simulink model "Dual_Active_Bridge_Converter"  (R2022b)
settings: Solver=ode23t  StartTime=0.0  StopTime=.1  FixedStep=1e-7  MaxStep=1e-7  RelTol=1e-3
model workspace (MAT data in the model file):
  N_P0 = 3
undefined symbols (not defined in the file or in its folder): Ion, Lithium
libraries: spsIGBTDiodeLib x8, spsCurrentMeasurementLib x3, spsVoltageMeasurementLib x3, spsSeriesRLCBranchLib x2, slpidlib x2, spsBatteryLib x1, spsDCVoltageSourceLib x1, spsLinearTransformerLib x1, dspstat3 x1, sps_lib x1
settings Model: Creator=es-ahmedabdellatif20  LastModifiedBy=es-ahmedabdellatif20

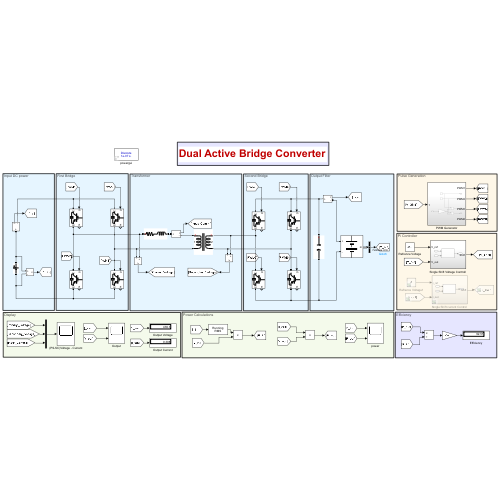
[thumbnail: Simulink's stored preview of the top-level diagram]
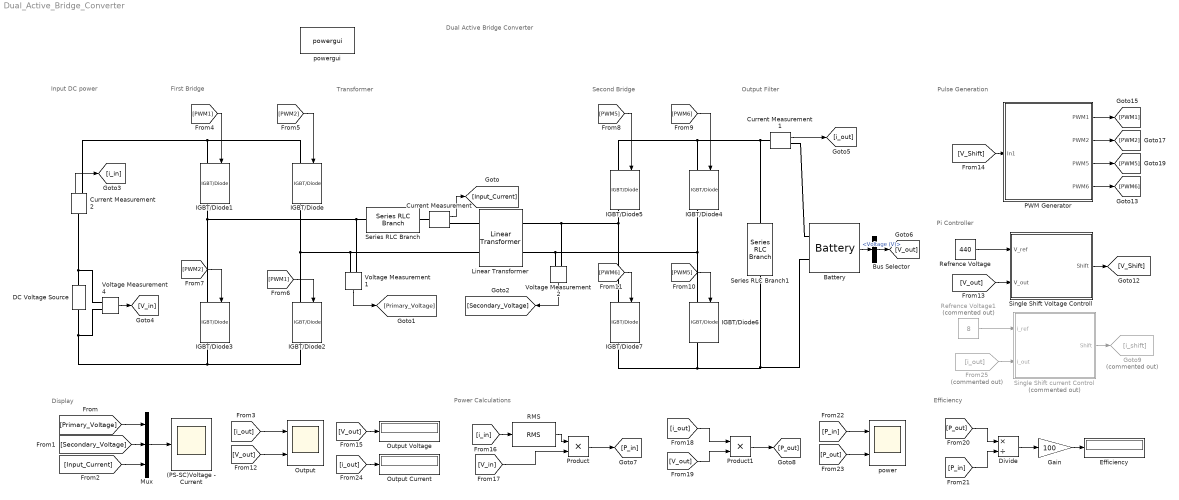
== system Dual_Active_Bridge_Converter ==
  note: Efficiency
  note: Power Calculations
  note: Pi Controller
  note: Pulse Generation
  note: Output Filter
  note: Second Bridge
  note: Transformer
  note: First Bridge
  note: Input DC power
  note: Dual Active Bridge Converter
  note: Display
  (PS-SC)Voltage - Current : Scope
  Battery : spsBatteryLib/Battery  BatType=Lithium-Ion  ShowTempParam=off  ThermalPreset=no  ShowAgeParam=off  NomV=400  NomQ=5  SOC=60  Batt_Tr=30  PresetModel=on  MaxQ=5  MinV=300  FullV=465.5949  Dis_rate=2.1739  R=0.8  Normal_OP=4.5217  expZone="[432.1543     0.2456522]"  current=[6.5 13 32.5]  Units=Time  Tci=20  NomT=20  T2=-30  MaxQ2=4.8  FullV2=7.1  Normal_OP2=5.655  expZone2="[6.58           1]"  Rca=0.6  ti=2000  Dp=0  Neq0=0  Tsim=1e6  Ta1=25  Qeol=5.4*0.9  Reol=0.013333*1.2  Char_age=[2.3478, 3]  Dis_age=[2.3478, 10]  N1=1500  N2=10500  N3=1000  N4=1400  Ta2=45  N5=950
  Bus Selector : BusSelector  OutputSignals=Voltage (V)
  Current Measurement : spsCurrentMeasurementLib/Current Measurement  PhasorSimulation=off  OutputType=Complex  PSBequivalent=0
  Current Measurement1 : spsCurrentMeasurementLib/Current Measurement  PhasorSimulation=off  OutputType=Complex  PSBequivalent=0
  Current Measurement2 : spsCurrentMeasurementLib/Current Measurement  PhasorSimulation=off  OutputType=Complex  PSBequivalent=0
  DC Voltage Source : spsDCVoltageSourceLib/DC Voltage Source  Amplitude=800  Measurements=Voltage
  Divide : Product  Inputs=*/
  Efficiency : Display
  From25 : From  Commented=on  GotoTag=i_out
  Gain : Gain  Gain=100
  Goto9 : Goto  Commented=on  GotoTag=i_shift
  IGBT/Diode{,1..7} (8 alike) : spsIGBTDiodeLib/IGBT//Diode  Ron=1e-3  Rs=1e5  Cs=inf  Measurements=on
  Linear Transformer : spsLinearTransformerLib/Linear Transformer  UNITS=SI  NominalPower=[ 10000 100000 ]  winding1=[800 0 0]  winding2=[450 0 0]  ThreeWindings=off  winding3=[3.15e+05 0.7938 0.084225]  RmLm=[1.0804e+06 2866]  Measurements=None  DataType=on
  Mux : Mux  Inputs=3
  Output : Scope  NumInputPorts=2
  Output Current : Display
  Output Voltage : Display
  PWM Generator : Subsystem
  Product : Product
  Product1 : Product
  RMS : dspstat3/RMS  run=on  directionMode=Each column  dimension=1  InputProcessing=Columns as channels (frame based)  reset_popup=None
  Refrence Voltage : Constant  Value=440
  Refrence Voltage1 : Constant  Commented=on  Value=8
  Series RLC Branch : spsSeriesRLCBranchLib/Series RLC Branch  LConnTagsString=__new0  RConnTagsString=__new0  BranchType=RL  Resistance=.2  Inductance=8.5e-5/2  SetiL0=off  InitialCurrent=5  Capacitance=1e-6  Setx0=off  InitialVoltage=0  Measurements=None
  Series RLC Branch1 : spsSeriesRLCBranchLib/Series RLC Branch  LConnTagsString=__new0  RConnTagsString=__new0  BranchType=C  Resistance=10  Inductance=2.2857e-4  SetiL0=off  InitialCurrent=0  Capacitance=660e-6  Setx0=on  InitialVoltage=250  Measurements=None
  "Single Shift Voltage Controll " : Subsystem
  "Single Shift current Control " : Subsystem  Commented=on
  Voltage Measurement1 : spsVoltageMeasurementLib/Voltage Measurement  PhasorSimulation=off  OutputType=Complex  PSBequivalent=0
  Voltage Measurement2 : spsVoltageMeasurementLib/Voltage Measurement  PhasorSimulation=off  OutputType=Complex  PSBequivalent=0
  Voltage Measurement4 : spsVoltageMeasurementLib/Voltage Measurement  PhasorSimulation=off  OutputType=Complex  PSBequivalent=0
  power : Scope  NumInputPorts=2
  powergui : sps_lib/powergui  Priority=1  SimulationMode=Discrete  SampleTime=1e-7  frequency=60  Iterations=50  frequencyindice=0  Pbase=100e6  ErrMax=1e-4  UnitsV=kV  UnitsW=MW  buscounter=0  FunctionMessages=off  echomessages=off  EnableUseOfTLC=off  CurrentSourceSwitches=off  DisableSnubberDevices=off  DisableRonSwitches=off  DisableVfSwitches=off  DisplayEquations=off  AutomaticDiscreteSolvers=off  SolverType=Tustin/Backward Euler (TBE)  Interpol=off  ExternalGateDelay=off  methode=off  Ts=100  x0status=blocks  SPID=on  SwTol=0  HookPort=off  NonlinearTolerance=1e-4  nMaxIteration=100  ContinueOnMaxIteration=off  RestoreLinks=warning  ResistiveCurrentMeasurement=off  Frange=[0:2:500]  Ylog=off  Xlog=on  ShowGrid=off  save=off  variable=ZData  structure=0  ZoomFFT=off  StartTime=0.0  cycles=1  DisplayStyle=1  fundamental=60  FreqAxis=off  MaxFrequency=1000  frequencyindicesteady=1  RmsSteady=1  display=off
  wires:
  Mux/1 -> (PS-SC)Voltage - Current/1
  Current Measurement/1 -> [Input_Current]
  Voltage Measurement1/1 -> [Primary_Voltage]
  Voltage Measurement2/1 -> [Secondary_Voltage]
  [Primary_Voltage] -> Mux/1
  [Secondary_Voltage] -> Mux/2
  [PWM1] -> IGBT/Diode1/1
  [PWM2] -> IGBT/Diode/1
  [PWM2] -> IGBT/Diode3/1
  [PWM1] -> IGBT/Diode2/1
  [PWM5] -> IGBT/Diode6/1
  [PWM6] -> IGBT/Diode4/1
  [PWM5] -> IGBT/Diode5/1
  [PWM6] -> IGBT/Diode7/1
  PWM Generator/1(PWM1) -> [PWM1]
  PWM Generator/2(PWM2) -> [PWM2]
  PWM Generator/3(PWM5) -> [PWM5]
  PWM Generator/4(PWM6) -> [PWM6]
  [Input_Current] -> Mux/3
  [V_Shift] -> PWM Generator/1(In1)
  Current Measurement1/1 -> [i_out]
  [V_out] -> "Single Shift Voltage Controll "/2(V_out)
  "Single Shift Voltage Controll "/1(Shift) -> [V_Shift]
  Refrence Voltage/1 -> "Single Shift Voltage Controll "/1(V_ref)
  [i_out] -> Output/1
  [V_out] -> Output/2
  [V_out] -> Output Voltage/1
  Current Measurement2/1 -> [i_in]
  Voltage Measurement4/1 -> [V_in]
  [i_out] -> Product1/1
  [V_out] -> Product1/2
  Product1/1 -> [P_out]
  [P_out] -> Divide/1
  [P_in] -> Divide/2
  Divide/1 -> Gain/1
  Gain/1 -> Efficiency/1
  [P_in] -> power/1
  [P_out] -> power/2
  [i_out] -> Output Current/1
  Battery/1 -> Bus Selector/1
  Refrence Voltage1/1 -> "Single Shift current Control "/1(i_ref)
  "Single Shift current Control "/1(Shift) -> Goto9/1
  From25/1 -> "Single Shift current Control "/2(i_out)
  Product/1 -> [P_in]
  RMS/1 -> Product/1
  [i_in] -> RMS/1
  [V_in] -> Product/2
  Bus Selector/1 -> [V_out]  "<Voltage (V)>"
  connections:
  IGBT/Diode3/LConn1 -- Series RLC Branch/LConn1 -- Voltage Measurement1/LConn1 -- IGBT/Diode1/RConn1
  IGBT/Diode2/LConn1 -- Linear Transformer/LConn2 -- Voltage Measurement1/LConn2 -- IGBT/Diode/RConn1
  IGBT/Diode2/RConn1 -- DC Voltage Source/LConn1 -- Voltage Measurement4/LConn2 -- IGBT/Diode3/RConn1
  Series RLC Branch/RConn1 -- Current Measurement/LConn1
  IGBT/Diode4/LConn1 -- Current Measurement1/LConn1 -- Series RLC Branch1/LConn1 -- IGBT/Diode5/LConn1
  IGBT/Diode6/LConn1 -- Linear Transformer/RConn2 -- Voltage Measurement2/LConn2 -- IGBT/Diode4/RConn1
  IGBT/Diode7/LConn1 -- IGBT/Diode5/RConn1 -- Linear Transformer/RConn1 -- Voltage Measurement2/LConn1
  IGBT/Diode6/RConn1 -- Battery/LConn2 -- Series RLC Branch1/RConn1 -- IGBT/Diode7/RConn1
  Current Measurement/RConn1 -- Linear Transformer/LConn1
  IGBT/Diode/LConn1 -- Current Measurement2/RConn1 -- IGBT/Diode1/LConn1
  DC Voltage Source/RConn1 -- Current Measurement2/LConn1 -- Voltage Measurement4/LConn1
  Current Measurement1/RConn1 -- Battery/LConn1

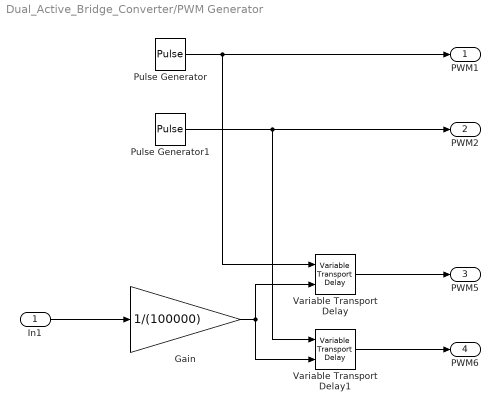
== system Dual_Active_Bridge_Converter/PWM Generator ==
  In1 : Inport
  Gain : Gain  Gain=1/(100000)
  Pulse Generator : DiscretePulseGenerator  PulseType=Time based  Period=1/(100000)  PulseWidth=49  PhaseDelay=5e-8
  Pulse Generator1 : DiscretePulseGenerator  PulseType=Time based  Period=1/(100000)  PulseWidth=49  PhaseDelay=5.05e-6
  Variable Transport Delay : VariableTransportDelay  VariableDelayType=Variable transport delay  MaximumDelay=10  MaximumPoints=500000
  Variable Transport Delay1 : VariableTransportDelay  VariableDelayType=Variable transport delay  MaximumDelay=10  MaximumPoints=400384
  PWM1 : Outport
  PWM2 : Outport  Port=2
  PWM5 : Outport  Port=3
  PWM6 : Outport  Port=4
  wires:
  Pulse Generator1/1 -> PWM2/1, Variable Transport Delay1/1
  Gain/1 -> Variable Transport Delay1/2, Variable Transport Delay/2
  Pulse Generator/1 -> PWM1/1, Variable Transport Delay/1
  Variable Transport Delay/1 -> PWM5/1
  Variable Transport Delay1/1 -> PWM6/1
  In1/1 -> Gain/1

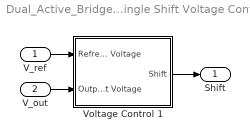
== system Dual_Active_Bridge_Converter/Single Shift Voltage Controll  ==
  V_ref : Inport
  V_out : Inport  Port=2
  Voltage Control 1 : Subsystem
  Shift : Outport
  wires:
  V_out/1 -> Voltage Control 1/2(Output Voltage)
  Voltage Control 1/1(Shift) -> Shift/1
  V_ref/1 -> Voltage Control 1/1(Refrence Voltage)

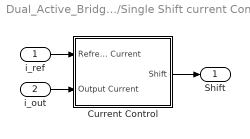
== system Dual_Active_Bridge_Converter/Single Shift current Control  ==
  i_ref : Inport
  i_out : Inport  Port=2
  "Current Control " : Subsystem
  Shift : Outport
  wires:
  i_ref/1 -> "Current Control "/1(Refrence Current)
  "Current Control "/1(Shift) -> Shift/1
  i_out/1 -> "Current Control "/2(Output Current)

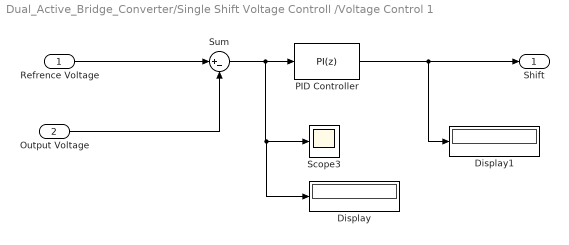
== system Dual_Active_Bridge_Converter/Single Shift Voltage Controll /Voltage Control 1 ==
  Refrence Voltage : Inport
  Output Voltage : Inport  Port=2
  Display : Display
  Display1 : Display
  PID Controller : slpidlib/PID Controller  Controller=PI  Form=Parallel  TimeDomain=Discrete-time  UseExternalTs=off  SampleTime=1e-7  IntegratorMethod=Forward Euler  FilterMethod=Forward Euler  ControllerParametersSource=internal  P=.000085  I=.25  UseKiTs=off  D=0  N=100  UseFilter=on  TunerSelectOption=Transfer Function Based (PID Tuner App)  InitialConditionSource=internal  InitialConditionForIntegrator=0  InitialConditionForFilter=0  DifferentiatorICPrevScaledInput=0  ExternalReset=none  TrackingMode=off  Kt=1  LimitOutput=on  SatLimitsSource=internal  UpperSaturationLimit=.035  LowerSaturationLimit=-.035  LinearizeAsGain=on  AntiWindupMode=clamping  Kb=1  LimitIntegrator=off  UpperIntegratorSaturationLimit=inf  LowerIntegratorSaturationLimit=-inf  POutMin=[]  POutMax=[]  IOutMin=[]  IOutMax=[]  DOutMin=[]  DOutMax=[]  NOutMin=[]  NOutMax=[]  SumOutMin=[]  SumOutMax=[]  SaturationOutMin=[]  SaturationOutMax=[]  PParamMin=[]  PParamMax=[]  IParamMin=[]  IParamMax=[]  DParamMin=[]  DParamMax=[]  NParamMin=[]  NParamMax=[]  KbParamMin=[]  KbParamMax=[]  KtParamMin=[]  KtParamMax=[]  KbOutMin=[]  KbOutMax=[]  KtOutMin=[]  KtOutMax=[]  IntegratorOutMin=[]  IntegratorOutMax=[]  FilterOutMin=[]  FilterOutMax=[]  SumI1OutMin=[]  SumI1OutMax=[]  SumI2OutMin=[]  SumI2OutMax=[]  SumI3OutMin=[]  SumI3OutMax=[]  SumI4OutMin=[]  SumI4OutMax=[]  SumDOutMin=[]  SumDOutMax=[]  DifferentiatorOutMin=[]  DifferentiatorOutMax=[]  FilterDiffOutCoefMin=[]  FilterDiffOutCoefMax=[]  ReciprocalOutMin=[]  ReciprocalOutMax=[]  SumDenOutMin=[]  SumDenOutMax=[]  SumNumOutMin=[]  SumNumOutMax=[]  DivideOutMin=[]  DivideOutMax=[]  UdiffTsProdOutMin=[]  UdiffTsProdOutMax=[]  NTsProdOutMin=[]  NTsProdOutMax=[]  UintegralTsProdOutMin=[]  UintegralTsProdOutMax=[]  UngainTsProdOutMin=[]  UngainTsProdOutMax=[]  ClampingZeroOutDataTypeStr=Inherit: Inherit via back propagation  ClampingZeroOutMin=[]  ClampingZeroOutMax=[]  FilterDenConstantOutDataTypeStr=Inherit: Inherit via back propagation  FilterDenConstantOutMin=[]  FilterDenConstantOutMax=[]  PCopyOutDataTypeStr=Inherit: Inherit via back propagation  PCopyOutMin=[]  PCopyOutMax=[]  NCopyOutDataTypeStr=Inherit: Inherit via back propagation  NCopyOutMin=[]  NCopyOutMax=[]  IntegratorContinuousStateAttributes=''  IntegratorStateMustResolveToSignalObject=off  IntegratorRTWStateStorageClass=Auto  FilterContinuousStateAttributes=''  FilterStateMustResolveToSignalObject=off  FilterRTWStateStorageClass=Auto  ParallelPVariant=InternalParameters  IdealPVariant=Disabled  IVariant=InternalParameters  DVariant=Disabled  IntegratorVariant=Discrete  SatVariant=Enabled  AWVariant=DiscClampingParallel  PCopyVariant=Disabled  TRVariant=Disabled  FdbkBlocksVariant=Forward  IdealPFdbkVariant=Disabled  SatFdbkVariant=Disabled  DerivativeFilterVariant=Disabled  NVariant=Disabled  NCopyVariant=Disabled_SignalSpec  FilterICVariant=Disabled  IntegratorICVariant=InternalICs  ExternalResetVariant=Disabled  TRSumVariant=Passthrough  SumFdbkVariant=Disabled  SumVariant=Sum_PI  TsampFilterVariant=InternalTs  TsampNgainVariant=Passthrough  TsampIntegralVariant=Passthrough  ExternalSaturationOutDataTypeStr=Inherit: Same as second input
  Scope3 : Scope
  Sum : Sum  Inputs=|+-
  Shift : Outport
  wires:
  Sum/1 -> Display/1, Scope3/1, PID Controller/1
  Refrence Voltage/1 -> Sum/1
  PID Controller/1 -> Display1/1, Shift/1
  Output Voltage/1 -> Sum/2

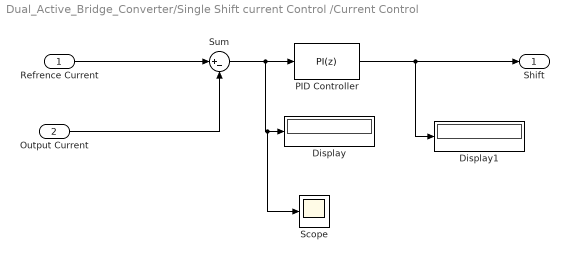
== system Dual_Active_Bridge_Converter/Single Shift current Control /Current Control  ==
  Refrence Current : Inport
  Output Current : Inport  Port=2
  Display : Display
  Display1 : Display
  PID Controller : slpidlib/PID Controller  Controller=PI  Form=Parallel  TimeDomain=Discrete-time  UseExternalTs=off  SampleTime=1e-7  IntegratorMethod=Forward Euler  FilterMethod=Forward Euler  ControllerParametersSource=internal  P=.00025  I=10  UseKiTs=off  D=0  N=100  UseFilter=on  TunerSelectOption=Transfer Function Based (PID Tuner App)  InitialConditionSource=internal  InitialConditionForIntegrator=0  InitialConditionForFilter=0  DifferentiatorICPrevScaledInput=0  ExternalReset=none  TrackingMode=off  Kt=1  LimitOutput=on  SatLimitsSource=internal  UpperSaturationLimit=.035  LowerSaturationLimit=-.035  LinearizeAsGain=on  AntiWindupMode=clamping  Kb=1  LimitIntegrator=off  UpperIntegratorSaturationLimit=inf  LowerIntegratorSaturationLimit=-inf  POutMin=[]  POutMax=[]  IOutMin=[]  IOutMax=[]  DOutMin=[]  DOutMax=[]  NOutMin=[]  NOutMax=[]  SumOutMin=[]  SumOutMax=[]  SaturationOutMin=[]  SaturationOutMax=[]  PParamMin=[]  PParamMax=[]  IParamMin=[]  IParamMax=[]  DParamMin=[]  DParamMax=[]  NParamMin=[]  NParamMax=[]  KbParamMin=[]  KbParamMax=[]  KtParamMin=[]  KtParamMax=[]  KbOutMin=[]  KbOutMax=[]  KtOutMin=[]  KtOutMax=[]  IntegratorOutMin=[]  IntegratorOutMax=[]  FilterOutMin=[]  FilterOutMax=[]  SumI1OutMin=[]  SumI1OutMax=[]  SumI2OutMin=[]  SumI2OutMax=[]  SumI3OutMin=[]  SumI3OutMax=[]  SumI4OutMin=[]  SumI4OutMax=[]  SumDOutMin=[]  SumDOutMax=[]  DifferentiatorOutMin=[]  DifferentiatorOutMax=[]  FilterDiffOutCoefMin=[]  FilterDiffOutCoefMax=[]  ReciprocalOutMin=[]  ReciprocalOutMax=[]  SumDenOutMin=[]  SumDenOutMax=[]  SumNumOutMin=[]  SumNumOutMax=[]  DivideOutMin=[]  DivideOutMax=[]  UdiffTsProdOutMin=[]  UdiffTsProdOutMax=[]  NTsProdOutMin=[]  NTsProdOutMax=[]  UintegralTsProdOutMin=[]  UintegralTsProdOutMax=[]  UngainTsProdOutMin=[]  UngainTsProdOutMax=[]  ClampingZeroOutDataTypeStr=Inherit: Inherit via back propagation  ClampingZeroOutMin=[]  ClampingZeroOutMax=[]  FilterDenConstantOutDataTypeStr=Inherit: Inherit via back propagation  FilterDenConstantOutMin=[]  FilterDenConstantOutMax=[]  PCopyOutDataTypeStr=Inherit: Inherit via back propagation  PCopyOutMin=[]  PCopyOutMax=[]  NCopyOutDataTypeStr=Inherit: Inherit via back propagation  NCopyOutMin=[]  NCopyOutMax=[]  IntegratorContinuousStateAttributes=''  IntegratorStateMustResolveToSignalObject=off  IntegratorRTWStateStorageClass=Auto  FilterContinuousStateAttributes=''  FilterStateMustResolveToSignalObject=off  FilterRTWStateStorageClass=Auto  ParallelPVariant=InternalParameters  IdealPVariant=Disabled  IVariant=InternalParameters  DVariant=Disabled  IntegratorVariant=Discrete  SatVariant=Enabled  AWVariant=DiscClampingParallel  PCopyVariant=Disabled  TRVariant=Disabled  FdbkBlocksVariant=Forward  IdealPFdbkVariant=Disabled  SatFdbkVariant=Disabled  DerivativeFilterVariant=Disabled  NVariant=Disabled  NCopyVariant=Disabled_SignalSpec  FilterICVariant=Disabled  IntegratorICVariant=InternalICs  ExternalResetVariant=Disabled  TRSumVariant=Passthrough  SumFdbkVariant=Disabled  SumVariant=Sum_PI  TsampFilterVariant=InternalTs  TsampNgainVariant=Passthrough  TsampIntegralVariant=Passthrough  ExternalSaturationOutDataTypeStr=Inherit: Same as second input
  Scope : Scope
  Sum : Sum  Inputs=|+-
  Shift : Outport
  wires:
  Output Current/1 -> Sum/2
  PID Controller/1 -> Display1/1, Shift/1
  Refrence Current/1 -> Sum/1
  Sum/1 -> PID Controller/1, Scope/1, Display/1
